simulink model "Divide_By_Zero"  (R2025b)
settings: Solver=FixedStepDiscrete  StartTime=0.0  StopTime=10.0  FixedStep=0.01  RelTol=1e-3
libraries: simulink x1
settings Model: Creator=soura  LastModifiedBy=soura

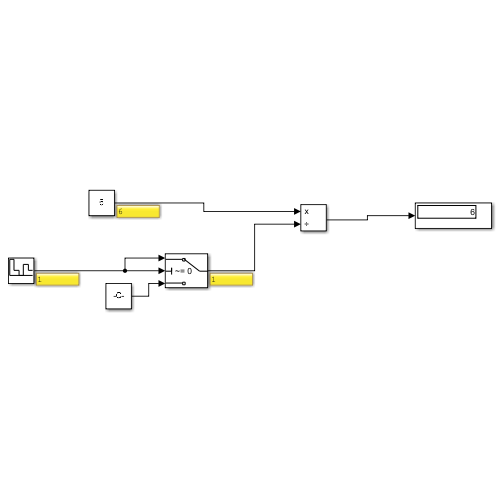
[thumbnail: Simulink's stored preview of the top-level diagram]
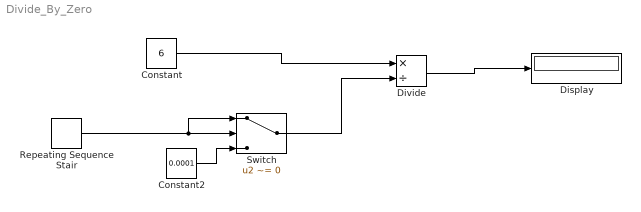
== system Divide_By_Zero ==
  Constant : Constant  Value=6
  Constant2 : Constant  Value=0.0001
  Display : Display
  Divide : Product  Inputs=*/
  Repeating Sequence Stair : simulink/Sources/Repeating Sequence Stair  OutValues=[3 1 0 2 1].'  tsamp=-1  OutMin=[]  OutMax=[]  OutDataTypeStr=double  OutputDataTypeScalingMode=double  OutDataType=fixdt(0,8)  ConRadixGroup=Best Precision: Vector-wise  OutScaling=2^-12
  Switch : Switch  Criteria=u2 ~= 0  SaturateOnIntegerOverflow=off  InputSameDT=off
  wires:
  Constant/1 -> Divide/1
  Repeating Sequence Stair/1 -> Switch/1, Switch/2
  Switch/1 -> Divide/2
  Divide/1 -> Display/1
  Constant2/1 -> Switch/3
